simulink model "sldemo_mdlref_conversion"  (Simulink 10.0)
settings: Solver=ode5  StartTime=0.0  StopTime=30  RelTol=1e-3  EnableMultiTasking=on
InitFcn:
  | warning('off','Simulink:Logging:DatasetRTWGenRootOutputNotSupported');
  | warning('off','Simulink:Logging:DatasetRTWGenStateNotSupported');
StartFcn:
  | warning('off','Simulink:Logging:DatasetRTWGenRootOutputNotSupported');
  | warning('off','Simulink:Logging:DatasetRTWGenStateNotSupported');
StopFcn:
  | warning('on','Simulink:Logging:DatasetRTWGenRootOutputNotSupported');
  | warning('on','Simulink:Logging:DatasetRTWGenStateNotSupported');
CloseFcn:
  | warning('on','Simulink:Logging:DatasetRTWGenRootOutputNotSupported');
  | warning('on','Simulink:Logging:DatasetRTWGenStateNotSupported');
PauseFcn:
  | warning('on','Simulink:Logging:DatasetRTWGenRootOutputNotSupported');
  | warning('on','Simulink:Logging:DatasetRTWGenStateNotSupported');
settings Model: Creator=The MathWorks, Inc.  ModifiedByFormat=The MathWorks Inc.  LastModifiedBy=The MathWorks Inc.  ExtModeAutoUpdateStatusClock=off
settings DataIOCC: LimitDataPoints=on  SaveFinalState=on  SaveFormat=Dataset  SaveState=on  SignalLoggingName=logsOut
settings OptimizationCC: DefaultParameterBehavior=Inlined  InlineInvariantSignals=on  ExpressionDepthLimit=2147483647  InitFltsAndDblsToZero=on
settings DebuggingCC: SaveWithParameterizedLinksMsg=none  UnderspecifiedInitializationDetection=Simplified  MergeDetectMultiDrivingBlocksExec=error  CheckExecutionContextPreStartOutputMsg=on  CheckExecutionContextRuntimeOutputMsg=on  MultiTaskDSMMsg=warning  MultiTaskCondExecSysMsg=none  SigSpecEnsureSampleTimeMsg=none  FcnCallInpInsideContextMsg=warning  RootOutportRequireBusObject=none  AllowSymbolicDim=off  StateNameClashWarn=warning  StrictBusMsg=ErrorOnBusTreatedAsVector
settings HardwareCC: TargetHWDeviceType=32-bit Generic
settings ModelReferenceCC: UpdateModelReferenceTargets=IfOutOfDate
settings CodeAppCC: MaxIdLength=100
settings GRTTargetCC: TargetFcnLib=ansi_tfl_tmw.mat  GeneratePreprocessorConditionals=Disable all
settings ConfigComp: CovExternalEMLEnable=off  CovSFcnEnable=off

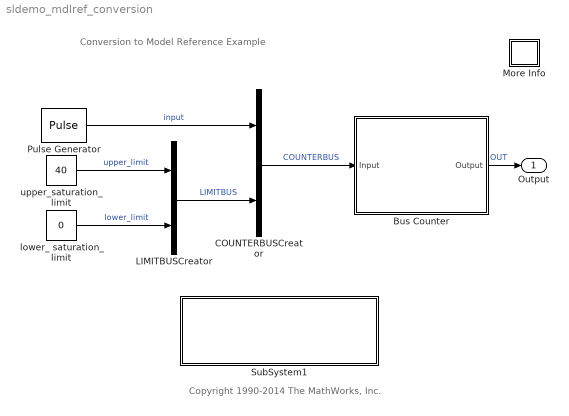
== system sldemo_mdlref_conversion ==
  note: Conversion to Model Reference Example
  note: Copyright 1990-2014 The MathWorks, Inc.
  Bus Counter : Subsystem  TreatAsAtomicUnit=on
  COUNTERBUSCreator : BusCreator  Inputs=2
  LIMITBUSCreator : BusCreator  Inputs=2
  More Info : Subsystem
      settings: OpenFcn=showdemo(bdroot(gcb))
      mask Display: disp('?')
  Pulse Generator : DiscretePulseGenerator  Amplitude=int32(1)  SampleTime=0.1
  SubSystem1 : Subsystem
      settings: OpenFcn=|
      | sldemo_mdlref_util('sldemo_mdlref_conversion','convert')
      | lasterror('reset')
      mask Display: disp('Double click here to convert \n ''Bus Counter'' Subsystem to \n Referenced Model');
  lower_ saturation_ limit : Constant  Value=0  OutDataTypeStr=int32  SampleTime=0.1
  upper_saturation_limit : Constant  Value=40  OutDataTypeStr=int32  SampleTime=0.1
  Output : Outport  VectorParamsAs1DForOutWhenUnconnected=off
  wires:
  upper_saturation_limit/1 -> LIMITBUSCreator/1  "upper_limit"
  lower_ saturation_ limit/1 -> LIMITBUSCreator/2  "lower_limit"
  LIMITBUSCreator/1 -> COUNTERBUSCreator/2  "LIMITBUS"
  COUNTERBUSCreator/1 -> Bus Counter/1(Input)  "COUNTERBUS"
  Bus Counter/1(Output) -> Output/1  "OUT"
  Pulse Generator/1 -> COUNTERBUSCreator/1  "input"

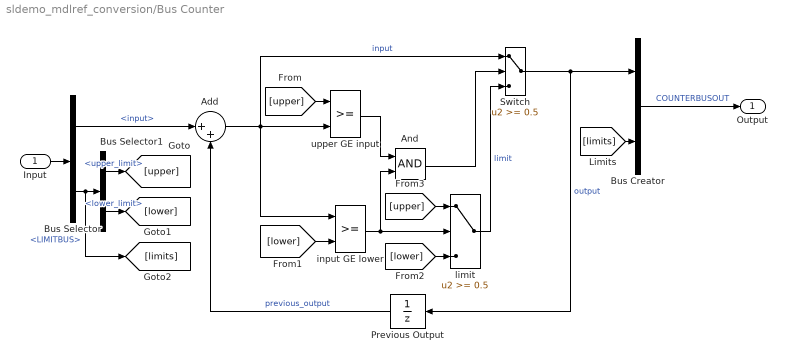
== system sldemo_mdlref_conversion/Bus Counter ==
  Input : Inport
  " input GE lower" : RelationalOperator  Priority=1  OutDataTypeStr=boolean  RndMeth=Nearest  InputSameDT=on
      settings: AttributesFormatString=\n
  " limit" : Switch  Threshold=0.5  SaturateOnIntegerOverflow=on  InputSameDT=on
  Add : Sum  Inputs=|++
  And : Logic  OutDataTypeStr=boolean
  Bus Creator : BusCreator  Inputs=2
  Bus Selector : BusSelector  OutputSignals=input,LIMITBUS
  Bus Selector1 : BusSelector  OutputSignals=upper_limit,lower_limit
  Previous Output : UnitDelay  SampleTime=-1  HasFrameUpgradeWarning=on
  Switch : Switch  Threshold=0.5  SaturateOnIntegerOverflow=on  InputSameDT=on
  upper GE input : RelationalOperator  Priority=0  OutDataTypeStr=boolean  RndMeth=Nearest  InputSameDT=on
      settings: AttributesFormatString=\n
  Output : Outport  VectorParamsAs1DForOutWhenUnconnected=off
  wires:
  [upper] -> " limit"/1
  Switch/1 -> Previous Output/1, Bus Creator/1  "output"
  " limit"/1 -> Switch/3  "limit"
  upper GE input/1 -> And/1
  Previous Output/1 -> Add/2  "previous_output"
  [lower] -> " limit"/3
  [upper] -> upper GE input/1
  [lower] -> " input GE lower"/2
  " input GE lower"/1 -> " limit"/2, And/2
  And/1 -> Switch/2
  Add/1 -> Switch/1, upper GE input/2, " input GE lower"/1  "input"
  Input/1 -> Bus Selector/1
  Bus Selector/2 -> [limits], Bus Selector1/1  "<LIMITBUS>"
  Bus Selector/1 -> Add/1  "<input>"
  Bus Selector1/1 -> [upper]  "<upper_limit>"
  Bus Selector1/2 -> [lower]  "<lower_limit>"
  Bus Creator/1 -> Output/1  "COUNTERBUSOUT"
  [limits] -> Bus Creator/2

== system sldemo_mdlref_conversion/More Info ==
  note: This demonstration shows how signals may be grouped and ungrouped while
      | retaining their names.  In this demonstration, 5 signals are created and labelled
      | appropriately.  These signals are then mux'd together to create a bus of signals.
      | This bus of signals is then fed into the Bus Selector block.  Inside of the Bus
      | Selector block, the Pulse and Chirp signals are chosen to be output from the
      | original signal bus.
      |
      | It is possible to place a nest signal buses and then still retrieve the original signal
      | with its label.
  note: Bus Block Demonstration

== system sldemo_mdlref_conversion/SubSystem1 ==
